simulink model "conjunto2TorqRods1RodaReacao"  (R2023b)
settings: Solver=FixedStepAuto  StartTime=0.0  StopTime=tf  FixedStep=step_modelo  RelTol=1e-3
undefined symbols (not defined in the file): B, IAU, Iw, Ixx, Iyy, Izz, Km, Kv, limCorrente, limVolt, Rm, RodKi, sat_rodareacao, sat_torquerod, torqrodAtivo, WMM2020
libraries: aerolibtransform2 x1, aerolibgravity2 x1
settings Model: PacingRate=1000  Creator=rodri  LastModifiedBy=rodri
settings DataIOCC: SaveOutput=off  SaveTime=off
settings DebuggingCC: ModelReferenceExtraNoncontSigs=warning

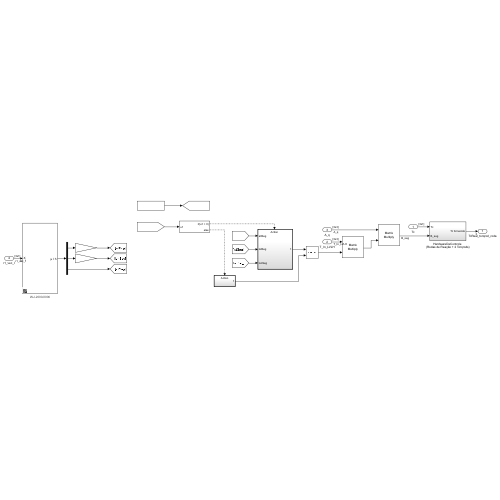
[thumbnail: Simulink's stored preview of the top-level diagram]
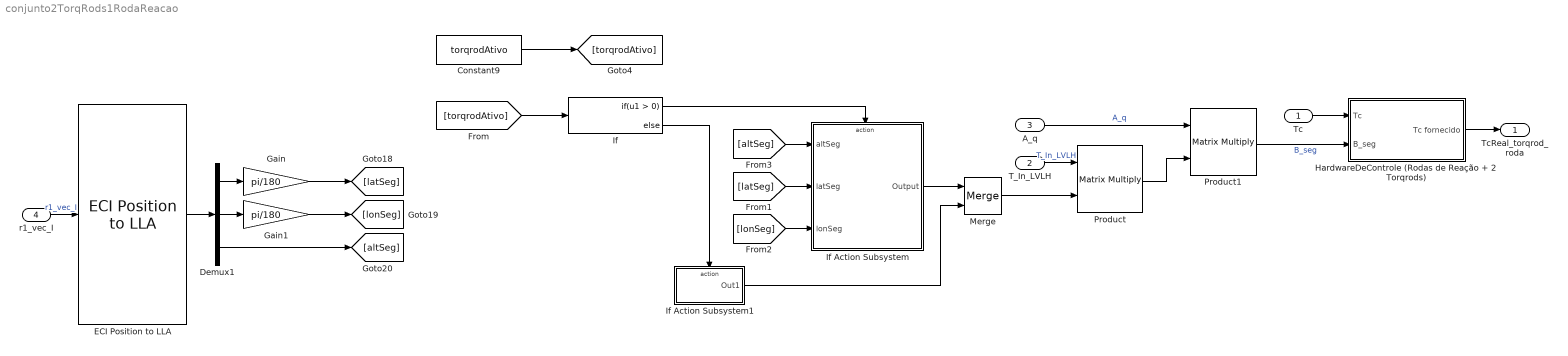
== system conjunto2TorqRods1RodaReacao ==
  Tc : Inport  OutDataTypeStr=double  PortDimensions=[3 1]  SampleTime=0
  T_In_LVLH : Inport  Port=2  OutDataTypeStr=double  PortDimensions=[3 3]  SampleTime=0
  A_q : Inport  Port=3  OutDataTypeStr=double  PortDimensions=[3 3]  SampleTime=0
  r1_vec_I : Inport  Port=4  OutDataTypeStr=double  PortDimensions=[3 1]  SampleTime=0
  Constant9 : Constant  Value=torqrodAtivo  SampleTime=-1
  Demux1 : Demux  Outputs=3
  ECI Position to LLA : aerolibtransform2/ECI Position to LLA  red=IAU-2000/2006  year=2013  month=January  day=1  hour=0  min=0  sec=0  deltaT=None  errorflag=Error  extraparamflag=off  eunits=Metric (MKS)  earthmodel=WGS84  flat=1/298.257223563  eqradius=6378137
      settings: AttributesFormatString=%<red>
  Gain : Gain  Gain=pi/180
  Gain1 : Gain  Gain=pi/180
  HardwareDeControle (Rodas de Reação + 2 Torqrods) : Subsystem
  If : If
  If Action Subsystem : Subsystem  TreatAsAtomicUnit=on
  If Action Subsystem1 : Subsystem  TreatAsAtomicUnit=on
  Merge : Merge
  Product : Product  Multiplication=Matrix(*)
  Product1 : Product  Multiplication=Matrix(*)
  TcReal_torqrod_roda : Outport  OutDataTypeStr=double  PortDimensions=3  SampleTime=0
  wires:
  HardwareDeControle (Rodas de Reação + 2 Torqrods)/1(Tc fornecido) -> TcReal_torqrod_roda/1
  Tc/1 -> HardwareDeControle (Rodas de Reação + 2 Torqrods)/1(Tc)
  T_In_LVLH/1 -> Product/1  "T_In_LVLH"
  Product/1 -> Product1/2
  Product1/1 -> HardwareDeControle (Rodas de Reação + 2 Torqrods)/2(B_seg)  "B_seg"
  A_q/1 -> Product1/1  "A_q"
  Constant9/1 -> [torqrodAtivo]
  [torqrodAtivo] -> If/1
  If/1 -> If Action Subsystem/Action
  [lonSeg] -> If Action Subsystem/3(lonSeg)
  [altSeg] -> If Action Subsystem/1(altSeg)
  [latSeg] -> If Action Subsystem/2(latSeg)
  If/2 -> If Action Subsystem1/Action
  If Action Subsystem/1(Output) -> Merge/1
  If Action Subsystem1/1(Out1) -> Merge/2
  Merge/1 -> Product/2
  Demux1/3 -> [altSeg]
  Gain1/1 -> [lonSeg]
  Demux1/2 -> Gain1/1
  Demux1/1 -> Gain/1
  ECI Position to LLA/1 -> Demux1/1
  Gain/1 -> [latSeg]
  r1_vec_I/1 -> ECI Position to LLA/1  "r1_vec_I"

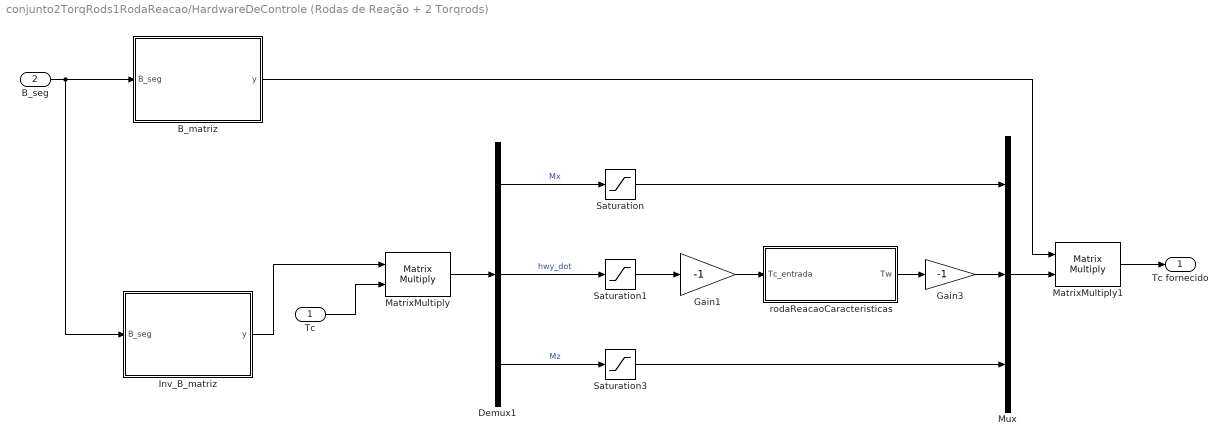
== system conjunto2TorqRods1RodaReacao/HardwareDeControle (Rodas de Reação + 2 Torqrods) ==
  Tc : Inport
  B_seg : Inport  Port=2
  B_matriz : MATLAB Function  TreatAsAtomicUnit=on
  Demux1 : Demux  Outputs=3
  Gain1 : Gain  Gain=-1
  Gain3 : Gain  Gain=-1
  Inv_B_matriz : MATLAB Function  TreatAsAtomicUnit=on
  MatrixMultiply : Product  Multiplication=Matrix(*)
  MatrixMultiply1 : Product  Multiplication=Matrix(*)
  Mux : Mux  Inputs=3
  Saturation : Saturate  UpperLimit=sat_torquerod  LowerLimit=-sat_torquerod
  Saturation1 : Saturate  UpperLimit=sat_rodareacao  LowerLimit=-sat_rodareacao
  Saturation3 : Saturate  UpperLimit=sat_torquerod  LowerLimit=-sat_torquerod
  rodaReacaoCaracteristicas : Subsystem
  Tc fornecido : Outport  VectorParamsAs1DForOutWhenUnconnected=off
  wires:
  Inv_B_matriz/1(y) -> MatrixMultiply/1
  Gain3/1 -> Mux/2
  rodaReacaoCaracteristicas/1(Tw) -> Gain3/1
  Gain1/1 -> rodaReacaoCaracteristicas/1(Tc_entrada)
  MatrixMultiply1/1 -> Tc fornecido/1
  Mux/1 -> MatrixMultiply1/2
  Saturation3/1 -> Mux/3
  Saturation1/1 -> Gain1/1
  Saturation/1 -> Mux/1
  Demux1/3 -> Saturation3/1  "Mz"
  Demux1/2 -> Saturation1/1  "hwy_dot"
  Demux1/1 -> Saturation/1  "Mx"
  MatrixMultiply/1 -> Demux1/1
  Tc/1 -> MatrixMultiply/2
  B_seg/1 -> B_matriz/1(B_seg), Inv_B_matriz/1(B_seg)
  B_matriz/1(y) -> MatrixMultiply1/1

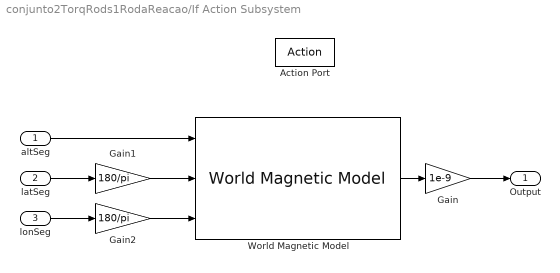
== system conjunto2TorqRods1RodaReacao/If Action Subsystem ==
  altSeg : Inport
  latSeg : Inport  Port=2
  lonSeg : Inport  Port=3
  Action Port : ActionPort
  Gain : Gain  Gain=1e-9
  Gain1 : Gain  Gain=180/pi
  Gain2 : Gain  Gain=180/pi
  World Magnetic Model : aerolibgravity2/World Magnetic Model  model=WMM2020 (2020-2025)  customFile='WMM2020.COF'  units=Metric (MKS)  time_in=off  month=January  day=1  year=2024  action=Error  h_out=off  dec_out=off  inc_out=off  ti_out=off
  Output : Outport
  wires:
  Gain2/1 -> World Magnetic Model/3
  World Magnetic Model/1 -> Gain/1
  latSeg/1 -> Gain1/1
  Gain1/1 -> World Magnetic Model/2
  lonSeg/1 -> Gain2/1
  altSeg/1 -> World Magnetic Model/1
  Gain/1 -> Output/1

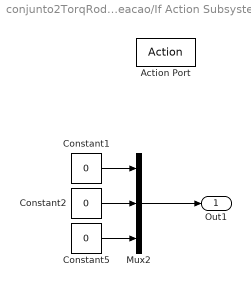
== system conjunto2TorqRods1RodaReacao/If Action Subsystem1 ==
  Action Port : ActionPort
  Constant1 : Constant  Value=0  SampleTime=-1
  Constant2 : Constant  Value=0  SampleTime=-1
  Constant5 : Constant  Value=0  SampleTime=-1
  Mux2 : Mux  Inputs=3
  Out1 : Outport
  wires:
  Constant2/1 -> Mux2/2
  Constant1/1 -> Mux2/1
  Mux2/1 -> Out1/1
  Constant5/1 -> Mux2/3

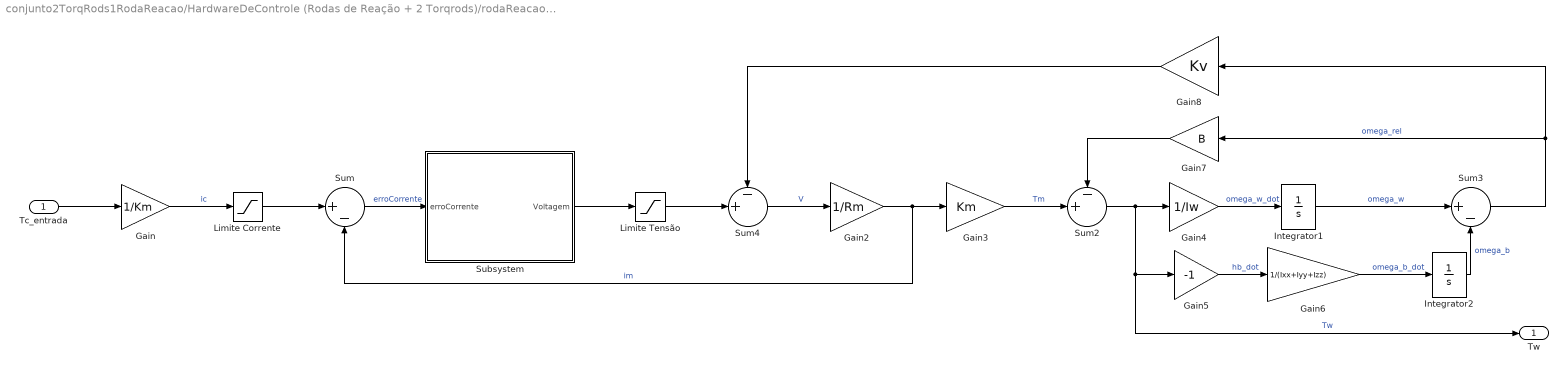
== system conjunto2TorqRods1RodaReacao/HardwareDeControle (Rodas de Reação + 2 Torqrods)/rodaReacaoCaracteristicas ==
  Tc_entrada : Inport
  Gain : Gain  Gain=1/Km
  Gain2 : Gain  Gain=1/Rm
  Gain3 : Gain  Gain=Km
  Gain4 : Gain  Gain=1/Iw
  Gain5 : Gain  Gain=-1
  Gain6 : Gain  Gain=1/(Ixx+Iyy+Izz)
  Gain7 : Gain  Gain=B
  Gain8 : Gain  Gain=Kv
  Integrator1 : Integrator
  Integrator2 : Integrator
  Limite Corrente : Saturate  UpperLimit=limCorrente  LowerLimit=-limCorrente
  Limite Tensão : Saturate  UpperLimit=limVolt  LowerLimit=-limVolt
  Subsystem : Subsystem
  Sum : Sum  Inputs=|+-
  Sum2 : Sum  Inputs=-+|
  Sum3 : Sum  Inputs=|+-
  Sum4 : Sum  Inputs=-+|
  Tw : Outport
  wires:
  Limite Tensão/1 -> Sum4/2
  Sum/1 -> Subsystem/1(erroCorrente)  "erroCorrente"
  Gain5/1 -> Gain6/1  "hb_dot"
  Gain6/1 -> Integrator2/1  "omega_b_dot"
  Gain8/1 -> Sum4/1
  Subsystem/1(Voltagem) -> Limite Tensão/1
  Gain/1 -> Limite Corrente/1  "ic"
  Tc_entrada/1 -> Gain/1
  Limite Corrente/1 -> Sum/1
  Gain7/1 -> Sum2/1
  Gain4/1 -> Integrator1/1  "omega_w_dot"
  Gain3/1 -> Sum2/2  "Tm"
  Integrator1/1 -> Sum3/1  "omega_w"
  Sum4/1 -> Gain2/1  "V"
  Gain2/1 -> Sum/2, Gain3/1  "im"
  Integrator2/1 -> Sum3/2  "omega_b"
  Sum3/1 -> Gain7/1, Gain8/1  "omega_rel"
  Sum2/1 -> Tw/1, Gain5/1, Gain4/1  "Tw"

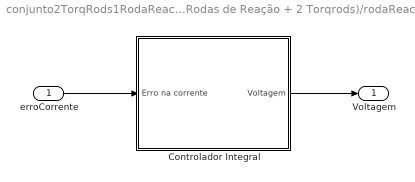
== system conjunto2TorqRods1RodaReacao/HardwareDeControle (Rodas de Reação + 2 Torqrods)/rodaReacaoCaracteristicas/Subsystem ==
  erroCorrente : Inport
  Controlador Integral : Subsystem
  Voltagem : Outport
  wires:
  erroCorrente/1 -> Controlador Integral/1(Erro na corrente)
  Controlador Integral/1(Voltagem) -> Voltagem/1

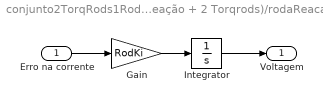
== system conjunto2TorqRods1RodaReacao/HardwareDeControle (Rodas de Reação + 2 Torqrods)/rodaReacaoCaracteristicas/Subsystem/Controlador Integral ==
  Erro na corrente : Inport
  Gain : Gain  Gain=RodKi
  Integrator : Integrator
  Voltagem : Outport  VectorParamsAs1DForOutWhenUnconnected=off
  wires:
  Integrator/1 -> Voltagem/1
  Erro na corrente/1 -> Gain/1
  Gain/1 -> Integrator/1

== matlab function conjunto2TorqRods1RodaReacao/HardwareDeControle (Rodas de Reação + 2 Torqrods)/Inv_B_matriz ==
  data: B_seg input; y output
function y = fcn(B_seg)

Bx = B_seg(1);
By = B_seg(2);
Bz = B_seg(3);

if By == 0
    y = [0 0 0; 0 0 0; 0 0 0];
else
    y = (1/(By^2))*[0 0 By
    Bx*By By^2 By*Bz
    -By 0 0];
end

== matlab function conjunto2TorqRods1RodaReacao/HardwareDeControle (Rodas de Reação + 2 Torqrods)/B_matriz ==
  data: B_seg input; y output
function y = fcn(B_seg)

Bx = B_seg(1);
By = B_seg(2);
Bz = B_seg(3);

y = [0 0 -By
    -Bz 1 Bx
    By 0 0];
